simulink model "gaetanprojs5"  (R2022b)
settings: Solver=FixedStepAuto  StartTime=0.0  StopTime=10.0  RelTol=1e-3  EnableMultiTasking=on
libraries: raspberrypiAVlib x4
settings Model: ExplicitPartitioning=on  Creator=tatan  LastModifiedBy=tatan
settings SolverCC: AllowMultiTaskInputOutput=on  ConcurrentTasks=on  PositivePriorityOrder=on  AutoInsertRateTranBlk=on
settings OptimizationCC: EnhancedBackFolding=on  PassReuseOutputArgsAs=Individual arguments  ZeroExternalMemoryAtStartup=off  ZeroInternalMemoryAtStartup=off  MaxStackSize=64  OptimizeBlockOrder=speed  DifferentSizesBufferReuse=on  OptimizationCustomize=off  EfficientTunableParamExpr=on
settings DebuggingCC: ParameterTunabilityLossMsg=error
settings HardwareCC: ProdBitPerPointer=32  ProdBitPerSizeT=32  ProdBitPerPtrDiffT=32  ProdLargestAtomicInteger=Long  ProdLargestAtomicFloat=Double  ProdWordSize=32  ProdLongLongMode=on  ProdHWDeviceType=ARM Compatible->ARM Cortex  UseEmbeddedCoderFeatures=off
settings RTWCC: Description=Embedded Coder  SystemTargetFile=ert.tlc  HardwareBoard=Raspberry Pi  TemplateMakefile=ert_default_tmf  Toolchain=GNU GCC Embedded Linux  BuildConfiguration=Faster Runs
settings CodeAppCC: ForceParamTrailComments=on  OperatorAnnotations=on  SimulinkDataObjDesc=on  SFDataObjDesc=on  InsertBlockDesc=on
settings ERTTargetCC: SupportNonInlinedSFcns=on  SupportVariableSizeSignals=on  ExtModeTransport=2  ExtModeStaticAlloc=on  ExtModeMexFile=ext_xcp  ExtModeMexArgs='10.0.4.203' 0 17725  ExtModeIntrfLevel=Level2 - Open  ERTSrcFileBannerTemplate=codertarget_code_template.cgt  ERTHdrFileBannerTemplate=codertarget_code_template.cgt  ERTDataSrcFileTemplate=codertarget_code_template.cgt  ERTDataHdrFileTemplate=codertarget_code_template.cgt

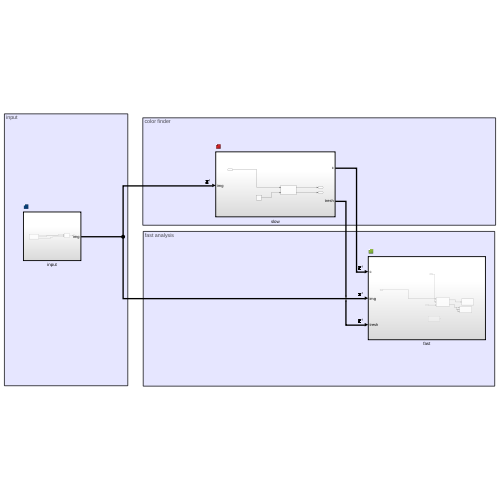
[thumbnail: Simulink's stored preview of the top-level diagram]
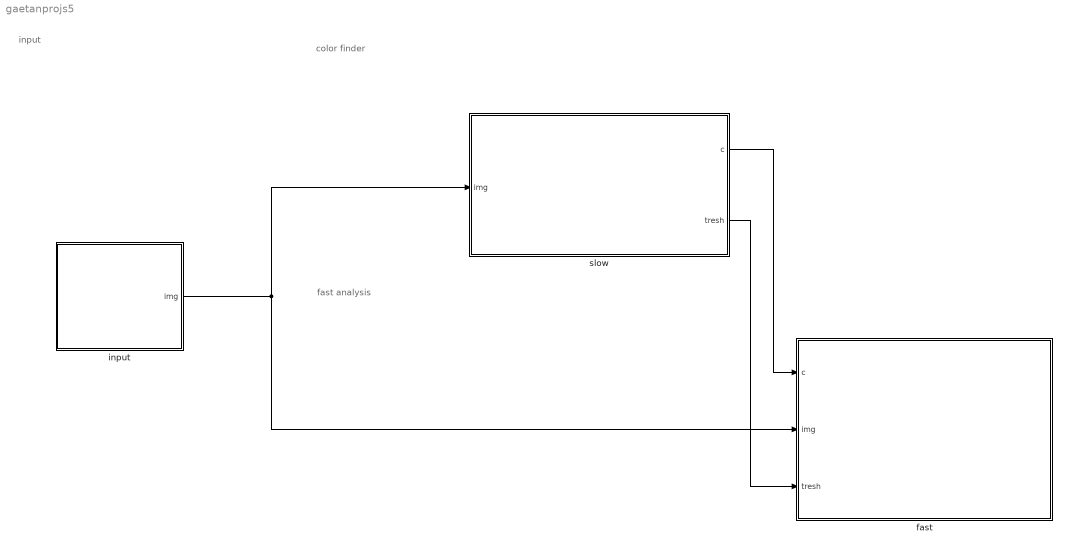
== system gaetanprojs5 ==
  note: input
  note: fast analysis
  note: color finder
  fast : Subsystem  TreatAsAtomicUnit=on
  input : Subsystem  TreatAsAtomicUnit=on
  slow : Subsystem  TreatAsAtomicUnit=on
  wires:
  slow/1(c) -> fast/1(c)
  input/1(img) -> fast/2(img), slow/1(img)
  slow/2(tresh) -> fast/3(tresh)

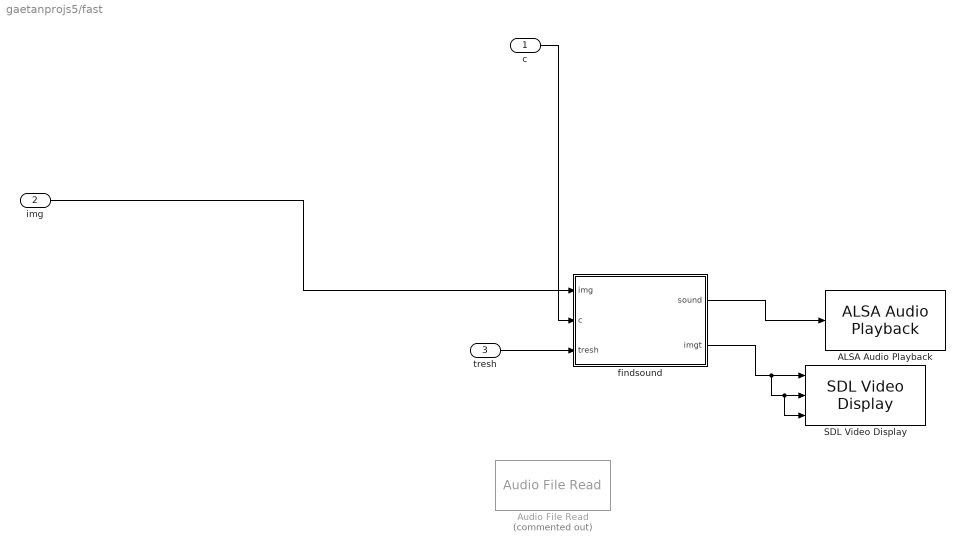
== system gaetanprojs5/fast ==
  c : Inport
  img : Inport  Port=2
  tresh : Inport  Port=3
  ALSA Audio Playback : raspberrypiAVlib/ALSA Audio Playback  deviceStr='plughw:0,0'  sampleRateEnum=44100  queueDuration=0.5  blockPlatform=LINUX
  Audio File Read : raspberrypiAVlib/Audio File Read  Commented=on  FileName=helicopter.wav  PlayCount=Inf  OutputEOFIndicator=off  SamplesPerFrame=4410
  SDL Video Display : raspberrypiAVlib/SDL Video Display  title=SDL Video Display  pixelFormat=RGB  pixelOrder=Planar  rowMajor=on  blockPlatform=Raspberry Pi
  findsound : MATLAB Function  TreatAsAtomicUnit=on
  wires:
  img/1 -> findsound/1(img)
  findsound/1(sound) -> ALSA Audio Playback/1
  c/1 -> findsound/2(c)
  tresh/1 -> findsound/3(tresh)
  findsound/2(imgt) -> SDL Video Display/3, SDL Video Display/2, SDL Video Display/1

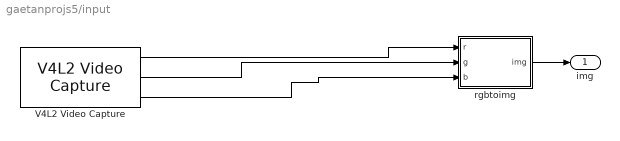
== system gaetanprojs5/input ==
  V4L2 Video Capture : raspberrypiAVlib/V4L2 Video Capture  DeviceName=/dev/video0  Resolution=320x240  CustomResolution=[ 320, 240 ]  PixelFormat=RGB  SampleTime=0.1  pixelOrder=planar  simOutput=Colorbars  imSizeSelection=320x240  imSize=[640, 480]  roi=[0, 0, 640, 480]  m_devName='/dev/video0'  blockPlatform=LINUX  HorizontalFlip=off  VerticalFlip=off  Brightness=0.5  Saturation=0.5  Contrast=0.5  Sharpness=0.5  CameraPan=0  CameraTilt=0  CameraZoom=0.5  EnableManualFocus=on  ManualFocus=0.5
  rgbtoimg : MATLAB Function  TreatAsAtomicUnit=on
  img : Outport
  wires:
  rgbtoimg/1(img) -> img/1
  V4L2 Video Capture/2 -> rgbtoimg/2(g)
  V4L2 Video Capture/1 -> rgbtoimg/1(r)
  V4L2 Video Capture/3 -> rgbtoimg/3(b)

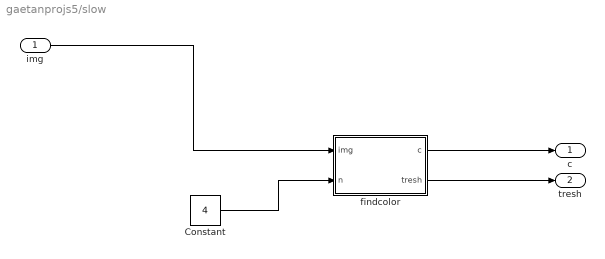
== system gaetanprojs5/slow ==
  img : Inport
  Constant : Constant  Value=4
  findcolor : MATLAB Function  TreatAsAtomicUnit=on
  c : Outport
  tresh : Outport  Port=2
  wires:
  Constant/1 -> findcolor/2(n)
  findcolor/1(c) -> c/1
  img/1 -> findcolor/1(img)
  findcolor/2(tresh) -> tresh/1

== matlab function gaetanprojs5/input/rgbtoimg ==
  data: r input; img output; g input; b input
function img= rgbtoimg(r,g,b)
    S = size(r);
    imgt=zeros(S(1,1),S(1,2),3);
    imgt(:,:,1) = r(:,:);
    imgt(:,:,2) = g(:,:);
    imgt(:,:,3) = b(:,:);
img = int8(imgt);

== matlab function gaetanprojs5/slow/findcolor ==
  data: img input; c output; n input; tresh output
function [c,tresh] = findcolor(img,n)
    [img,map,D] = quantize(img,n);
    map
    img;
    %imshow(img,map);
    
    index=1;
    minerror = regressionlineair(img,index);%the output of regression lineaire is actually a confidence statement
    minerror = minerror(1,3)
    for i=2:n
        therror = regressionlineair(img,i);
        therror = therror(1,3)
        if therror<minerror
            minerror = therror;
            index = i;
        end
    end
    index;
    D(:,index);
    ct = map(index,:);
    c = ct;
%   centroid = [];
%   S = size(img);
%     
%     for x=1:S(1,1)
%         for y=1:S(1,2)
%             if img(x,y)==index
%                 centroid = [ centroid, sqrt(D(x*y, index))];
%                 D(x*y,index);
%             end
%         end
%     end
%     centroid;
%     tresh = median(centroid);
    S = size(img);
    min = -1;
    for i=1:n
        if i~=index  
            for x=1:S(1,1)
                    for y=1:S(1,2)
                        if img(x,y)==i
                            if min ~= -1
                                if sqrt(D(x*y, i))<min
                                    min = sqrt(D(x*y, i));
                                end
                            end
                            min = sqrt(D(x*y, i));
                        end
                    end
            end
        end
    end
    tresh = min;
end

function coef = regressionlineair(img, i)
    S = size(img);
    Points = [];
    for l=1:S(1,1)
       Points = [ Points trouvermilieux(img,l,i)];
    end
    x = Points(1,:);
    x = transpose(x);
    s = size(x);
    un = ones(s(1,1),1);
    y = Points(2,:);
    y = transpose(y);
    x = double(x);
    y = double(y);
    [p,S] = polyfit(x,y,1);
    b = [p sum((y - p(1)*x+p(2)*ones(s)).^2)];
    coef = b;
end


function pix = trouvermilieux(img, l, i)
    S = size(img);
    c = 1;
    temp = [];
    while c<S(1,2)
        while img(l,c)~=i & c < S(1,2)
            c=c+1;
        end

        debut = c;
        while img(l,c)==i & c < S(1,2)
            c=c+1;
        end
        fin = int16(c-1);
        if img(l,debut)==i & img(l,fin)==i
            vec = [l int16((debut+fin)/2)];
            vec = transpose(vec);
            temp = [ temp vec];
        end
    end
    pix = temp;
end
% 
% function [img,map,D] = quantize(rgb,k)
% S=size(rgb);
% tmp = ones(3,S(1,1)*S(1,2));
% for l=1:S(1,1)
%     tmp(:,(l-1)*S(1,2)+1:l*S(1,2))=transpose(squeeze(rgb(l,:,:)));
% end
% [idx,C,sumd,D] = kmeans(transpose(tmp),k);
% idx;
% C;
% sumd;
% imgt = ones(S(1,1),S(1,2));
% 
% for i=1:S(1,1)*S(1,2)
%     imgt(uint32(i/S(1,2))+1,mod(i,S(1,2))+1) = idx(i);
% end
% size(imgt);
% %mapt = int32(C);
% imgt;
% imgt(S(1,1)+1,:) = [];
% %imgt = medfilt2(imgt,[8,8]);
% 
% img = uint8(imgt);
% map = uint8(C);
% end
% 

function [img,map,D] = quantize(rgb,k)
S=size(rgb);
tmp = ones(3,S(1,1)*S(1,2));
for l=1:S(1,1)
    tmp(:,(l-1)*S(1,2)+1:l*S(1,2))=transpose(squeeze(rgb(l,:,:)));
end
[idx,C,~,D] = kmeans(transpose(tmp),k);
imgt = ones(S(1,1),S(1,2));

for i=1:(S(1,1)-1)*S(1,2)
    imgt(uint32(i/S(1,2))+1,mod(i,S(1,2))+1) = idx(i);
end
size(imgt);
size(rgb);
%mapt = uint8(C);
%imgt(S(1,1)+1,:) = [];

%imgt = medfilt2(imgt,[8,8]);
%img = uint8(imgt);%%signe ici. Ne fonctionne qu'en double. Sinon il
%devient fou
img = imgt;
%map = uint8(C);%mieux vaut garder la precision
map = C;
end

== matlab function gaetanprojs5/fast/findsound ==
  data: img input; sound output; c input; tresh input; imgt output

function [sound,imgt] = findsound(img,c,tresh)
S = size(img);
for l=1:S(1,1)
    for x=1:S(1,2)
        tp=img(l,x,:);
        if manorm(double([tp(1),tp(2),tp(3)])-c(1,:))>tresh
            img(l,x,:) = [0,0,0];
        else
            img(l,x,:) = [255,255,255];
        end

    end
end

img = rgb2gray(uint8(img));
img = medfilt2(img,[16,16]);
%imshow(img)
imgt = img;
coef=regressionlineair(img);
% coef;
angle = ( atan(abs(coef)))*sign(coef);%angle * 180/pi, sens trigo
angle * 180/pi;
w = 440;%Hz
mono = linspace(0,1,44100);
mono = sin(mono*w);%comme ca en norme de stereo on retrouve mono
%mono = music;
%mono = mono.^2;
if angle > pi/4
   soundt = [zeros(1,44100);mono(1,:)];
elseif angle < -pi/4
   soundt = [mono(1,:);zeros(1,44100)];
else
   soundt = [mono(1,:)*sin((angle+pi/4));mono(1,:)*cos(angle+pi/4)];
end
%soundt;
sound = transpose(int16(65536*soundt));
%sound = soundt;
end


function coef = regressionlineair(img)
    S = size(img);
    Points = [];
    for l=1:S(1,1)
       Points = [ Points trouvermilieux(img,l)];
    end
    x = Points(1,:);
    x = transpose(x);
    s = size(x);
    un = ones(s(1,1),1);
    %x = [un x];
    y = Points(2,:);
    y = transpose(y);
    x = double(x);
    y = double(y);
    %[b, bint, r, rint, stats] = regress(y,x);
    p = polyfit(x,y,1);
    %stats
    %autcoef = regress(y,xe)
    %coef = x\y
    coef = p(1,1);
    %coef = 1
end


function pix = trouvermilieux(img, l)
    S = size(img);
    c = 1;
    temp = [];
    while c<S(1,2)
        while img(l,c,:)==0 & c < S(1,2)
            c=c+1;
        end

        debut = c;
        while img(l,c,:)>0 & c < S(1,2)
            c=c+1;
        end
        fin = int32(c-1);
        if c < S(1,2)
            vec = [l int32((debut+fin)/2)];
            vec = transpose(vec);
            temp = [ temp vec];
        end
        
    end
    pix = temp;
end

function v = manorm(u)
    v = sqrt(double(u(1,1).^2+u(1,2).^2+u(1,3).^2));
end
